simulink model "Fir_Filter"  (R2020b)
settings: Solver=VariableStepAuto  StartTime=0.0  StopTime=10.0  RelTol=1e-3
model workspace: external: MAT-File Gain_val.mat (data not in the file)
values from neighbouring files (symbols this model uses):
  a = 0.2178    [Gain_val.mat]
  b = 0.4356    [Gain_val.mat]
  c = 0.3523    [Gain_val.mat]
  d = 0.3927    [Gain_val.mat]
  freq = [100 1124 3956 6535 7898]    [Gain_val.mat]
settings Model: OrderedModelArguments=off  Creator=ankit  LastModifiedBy=ankit

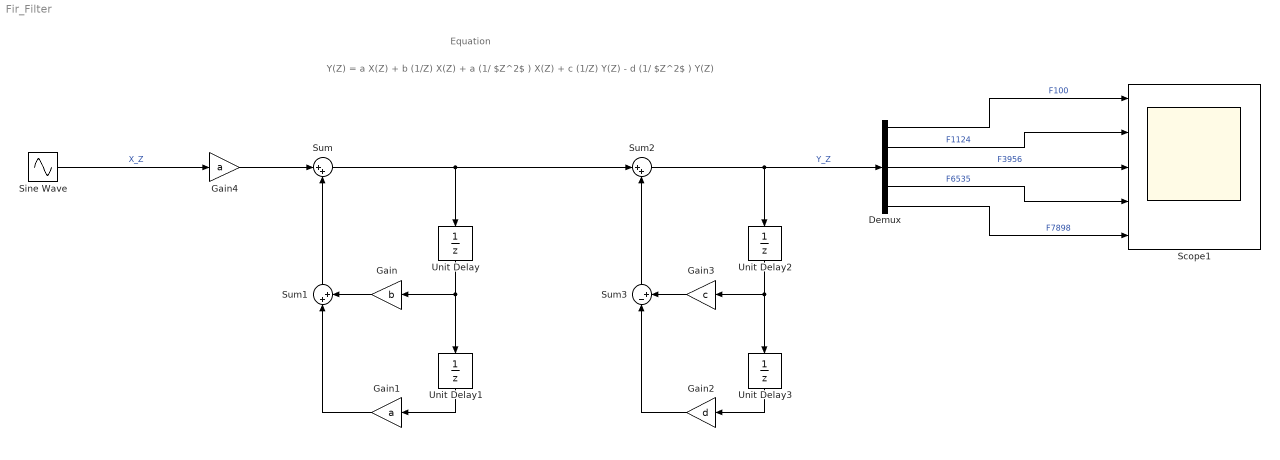
== system Fir_Filter ==
  note: Equation
  note: Y(Z) = a X(Z) + b (1/Z) X(Z) + a (1/ $Z^2$ ) X(Z) + c (1/Z) Y(Z) - d (1/ $Z^2$ ) Y(Z)
  Demux : Demux  Outputs=5
  Gain : Gain  Gain=b
  Gain1 : Gain  Gain=a
  Gain2 : Gain  Gain=d
  Gain3 : Gain  Gain=c
  Gain4 : Gain  Gain=a
  Scope1 : Scope  NumInputPorts=5
  Sine Wave : Sin  Frequency=freq  SampleTime=0
  Sum : Sum  Inputs=|++
  Sum1 : Sum  Inputs=|++
  Sum2 : Sum  Inputs=|++
  Sum3 : Sum  Inputs=|-+
  Unit Delay{,1..3} (4 alike) : UnitDelay  SampleTime=-1  HasFrameUpgradeWarning=on
  wires:
  Demux/1 -> Scope1/1  "F100"
  Demux/3 -> Scope1/3  "F3956"
  Unit Delay3/1 -> Gain2/1
  Unit Delay/1 -> Gain/1, Unit Delay1/1
  Unit Delay2/1 -> Unit Delay3/1, Gain3/1
  Unit Delay1/1 -> Gain1/1
  Sum2/1 -> Unit Delay2/1, Demux/1  "Y_Z"
  Sum3/1 -> Sum2/2
  Gain4/1 -> Sum/1
  Sum1/1 -> Sum/2
  Gain3/1 -> Sum3/2
  Demux/5 -> Scope1/5  "F7898"
  Sum/1 -> Sum2/1, Unit Delay/1
  Demux/2 -> Scope1/2  "F1124"
  Gain2/1 -> Sum3/1
  Gain1/1 -> Sum1/1
  Demux/4 -> Scope1/4  "F6535"
  Gain/1 -> Sum1/2
  Sine Wave/1 -> Gain4/1  "X_Z"
